simulink library "libreria_comunicaciones_red3"  (R2018a)
settings: Solver=VariableStepAuto  StartTime=0.0  StopTime=10.0  RelTol=1e-3
undefined symbols (not defined in the file or in its folder): Ts
settings Model: Creator=ana-n  LastModifiedBy=ana-n
settings CodeAppCC: StateflowObjectComments=on

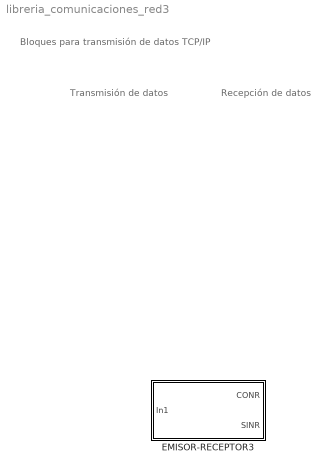
== system libreria_comunicaciones_red3 ==
  note: Bloques para transmisión de datos TCP/IP
  note: Recepción de datos
  note: Transmisión de datos
  EMISOR-RECEPTOR3 : Subsystem
      mask Display:
      | port_label('output',1,'CONR');
      | port_label('output',2,'SINR');
      | port_label('input',1,'Emisor');

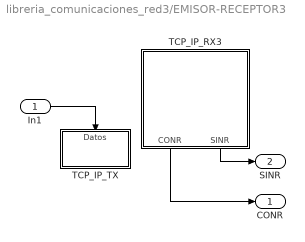
== system libreria_comunicaciones_red3/EMISOR-RECEPTOR3 ==
  In1 : Inport
  TCP_IP_RX3 : Subsystem
      mask Display:
      | disp('TCP_IP_RX')
      | port_label('output',1,'CONR');
      | port_label('output',2,'SINR');
  TCP_IP_TX : Subsystem
      mask Display: disp('TCP_IP_TX');
  CONR : Outport
  SINR : Outport  Port=2
  wires:
  TCP_IP_RX3/2(SINR) -> SINR/1
  TCP_IP_RX3/1(CONR) -> CONR/1
  In1/1 -> TCP_IP_TX/1(Datos)

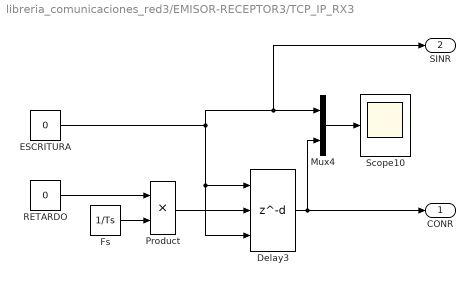
== system libreria_comunicaciones_red3/EMISOR-RECEPTOR3/TCP_IP_RX3 ==
  Delay3 : Delay  DelayLengthSource=Input port  DelayLength=1  DelayLengthUpperLimit=1000  InitialConditionSource=Input port  InitialCondition=0  InputProcessing=Inherited
      settings: InputPortMap=u0,p1,p4
  ESCRITURA : Constant  Value=0
  Fs : Constant  Value=1/Ts
  Mux4 : Mux  Inputs=2
  Product : Product
  RETARDO : Constant  Value=0
  Scope10 : Scope
  CONR : Outport
  SINR : Outport  Port=2
  wires:
  Mux4/1 -> Scope10/1
  ESCRITURA/1 -> Mux4/1, SINR/1, Delay3/1, Delay3/3
  Fs/1 -> Product/2
  RETARDO/1 -> Product/1
  Delay3/1 -> CONR/1, Mux4/2
  Product/1 -> Delay3/2

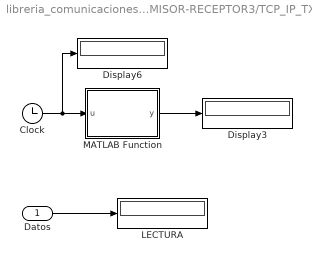
== system libreria_comunicaciones_red3/EMISOR-RECEPTOR3/TCP_IP_TX ==
  Datos : Inport
  Clock : Clock
  Display3 : Display
  Display6 : Display
  LECTURA : Display
  MATLAB Function : MATLAB Function  TreatAsAtomicUnit=on
  wires:
  Datos/1 -> LECTURA/1
  Clock/1 -> Display6/1, MATLAB Function/1(u)
  MATLAB Function/1(y) -> Display3/1

== matlab function libreria_comunicaciones_red3/EMISOR-RECEPTOR3/TCP_IP_TX/MATLAB Function ==
  data: u input; y output
%Esta función envía y recibos los datos
%desde el CCL a través del script_ciclo_vs.m
function y = fcn(u)
    coder.extrinsic('run')
    if mod(u,1/(60*32))==0 
        run script_ciclo_vs4.m
        y=1;
    else
        y=0;
    end
end
